simulink model "ultrasonictesting"  (R2024a)
settings: Solver=VariableStepAuto  StartTime=0.0  StopTime=10.0  RelTol=1e-3
libraries: dspsrcs4 x2, dspsigops x2, simulink_extras x1, dspswit3 x1
settings Model: Creator=felih  LastModifiedBy=felih

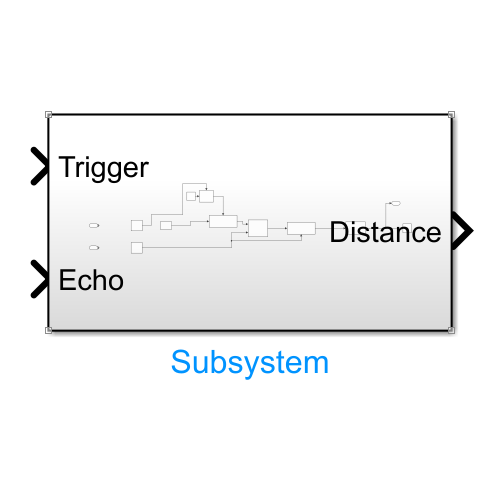
[thumbnail: Simulink's stored preview of the top-level diagram]
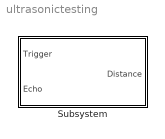
== system ultrasonictesting ==
  Subsystem : Subsystem

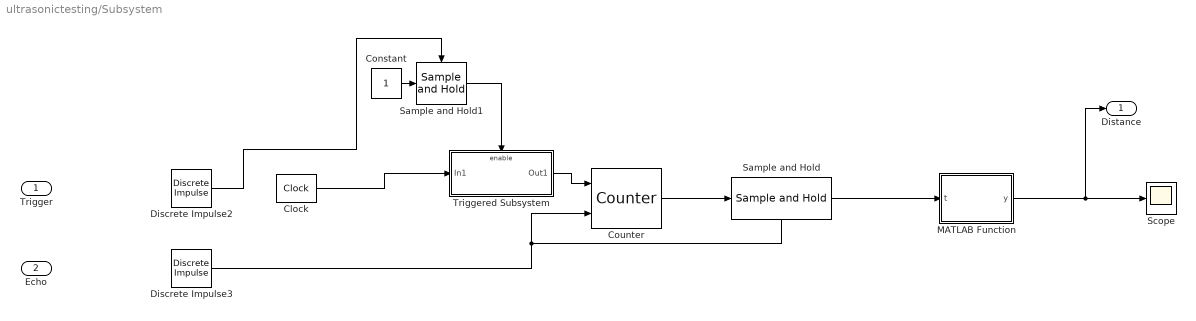
== system ultrasonictesting/Subsystem ==
  Trigger : Inport
  Echo : Inport  Port=2
  Clock : simulink_extras/Flip Flops/Clock  period=0.001
  Constant : Constant
  Counter : dspswit3/Counter  Direction=Up  CountEvent=Rising edge  CounterSize=32 bits  MaxCount=255  InitialCount=0  Output=Count  HitValue=32  ResetInput=on  SamplesPerFrame=1  Ts=1  CntDtype=double  HitDtype=Logical
  Discrete Impulse2 : dspsrcs4/Discrete  Impulse  Delay=1  SampleTime=0.001  FrameSample=1  OutputFrames=off  dataType=double  isSigned=on  wordLen=16  udDataType=sfix(16)  fracBitsMode=Best precision  numFracBits=15  OutDataTypeStr=double  LastOutDataTypeStr=double
  Discrete Impulse3 : dspsrcs4/Discrete  Impulse  Delay=2  SampleTime=1  FrameSample=1  OutputFrames=off  dataType=double  isSigned=on  wordLen=16  udDataType=sfix(16)  fracBitsMode=Best precision  numFracBits=15  OutDataTypeStr=double  LastOutDataTypeStr=double
  MATLAB Function : MATLAB Function  TreatAsAtomicUnit=on
  Sample and Hold : dspsigops/Sample and Hold  trig=Rising edge  initCond=0  latchinput=on
  Sample and Hold1 : dspsigops/Sample and Hold  trig=Rising edge  initCond=0  latchinput=off
  Scope : Scope
  Triggered Subsystem : Subsystem  TreatAsAtomicUnit=on
  Distance : Outport
  wires:
  Sample and Hold/1 -> MATLAB Function/1(t)
  Sample and Hold1/1 -> Triggered Subsystem/Enable
  Triggered Subsystem/1(Out1) -> Counter/1
  Discrete Impulse3/1 -> Sample and Hold/Trigger, Counter/2
  Discrete Impulse2/1 -> Sample and Hold1/Trigger
  Constant/1 -> Sample and Hold1/1
  Clock/1 -> Triggered Subsystem/1(In1)
  Counter/1 -> Sample and Hold/1
  MATLAB Function/1(y) -> Distance/1, Scope/1

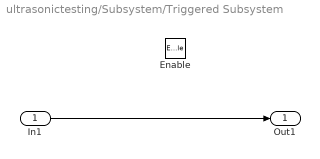
== system ultrasonictesting/Subsystem/Triggered Subsystem ==
  In1 : Inport
  Enable : EnablePort
  Out1 : Outport
  wires:
  In1/1 -> Out1/1

== matlab function ultrasonictesting/Subsystem/MATLAB Function ==
  data: t input; y output
function y = fcn(t)



y = ((t/1000)*340)/2;
